simulink subsystem "robotModel"  (R2022b)
settings: Solver=VariableStepAuto  StartTime=0.0  StopTime=10.0  RelTol=1e-3
undefined symbols (not defined in the file or in its folder): DiscIntNeverNeededParam
settings Model: Creator=Wikian  LastModifiedBy=Wikian

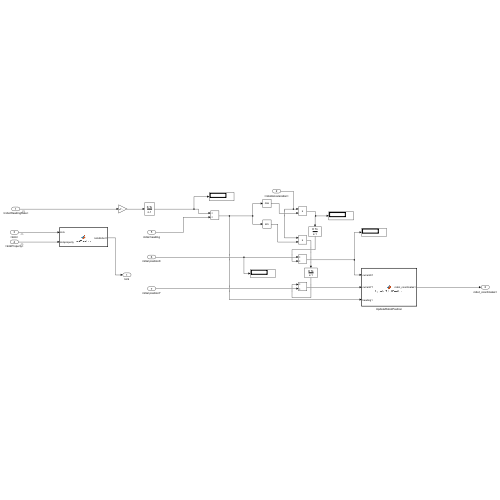
[thumbnail: Simulink's stored preview of the top-level diagram]
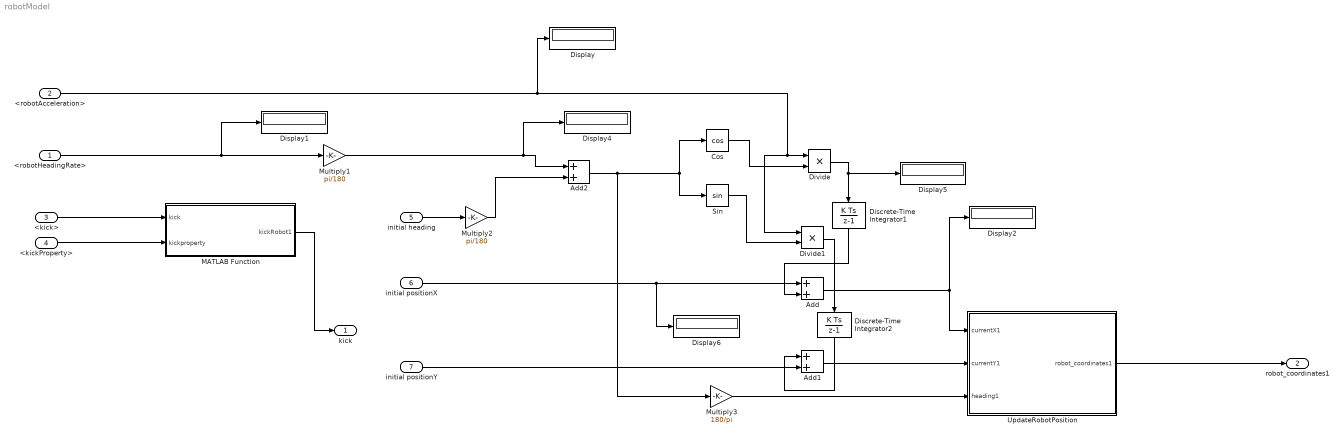
== system robotModel ==
  <robotHeadingRate> : Inport
  <robotAcceleration> : Inport  Port=2
  <kick> : Inport  Port=3
  <kickProperty> : Inport  Port=4
  initial heading : Inport  Port=5
  initial positionX : Inport  Port=6
  initial positionY : Inport  Port=7
  Add : Sum
  Add1 : Sum
  Add2 : Sum
  Cos : Trigonometry  Operator=cos
  Discrete-Time Integrator1 : DiscreteIntegrator  SampleTime=-1  ICPrevOutput=DiscIntNeverNeededParam  ICPrevScaledInput=DiscIntNeverNeededParam
  Discrete-Time Integrator2 : DiscreteIntegrator  SampleTime=-1  ICPrevOutput=DiscIntNeverNeededParam  ICPrevScaledInput=DiscIntNeverNeededParam
  Display{,1..2,4..6} (6 alike) : Display
  Divide : Product  Inputs=**
  Divide1 : Product  Inputs=**
  MATLAB Function : MATLAB Function  TreatAsAtomicUnit=on
  Multiply1 : Gain  Gain=pi/180
  Multiply2 : Gain  Gain=pi/180
  Multiply3 : Gain  Gain=180/pi
  Sin : Trigonometry
  UpdateRobotPosition : MATLAB Function  TreatAsAtomicUnit=on
  kick : Outport
  robot_coordinates1 : Outport  Port=2
  wires:
  Multiply2/1 -> Add2/2
  <robotHeadingRate>/1 -> Display1/1, Multiply1/1
  <kickProperty>/1 -> MATLAB Function/2(kickproperty)
  MATLAB Function/1(kickRobot1) -> kick/1
  <kick>/1 -> MATLAB Function/1(kick)
  Add/1 -> UpdateRobotPosition/1(currentX1), Display2/1
  UpdateRobotPosition/1(robot_coordinates1) -> robot_coordinates1/1
  Add1/1 -> UpdateRobotPosition/2(currentY1)
  initial positionX/1 -> Add/1, Display6/1
  initial positionY/1 -> Add1/2
  Sin/1 -> Divide1/2
  <robotAcceleration>/1 -> Display/1, Divide/1, Divide1/1
  Discrete-Time Integrator1/1 -> Add/2
  Divide1/1 -> Discrete-Time Integrator2/1
  Discrete-Time Integrator2/1 -> Add1/1
  initial heading/1 -> Multiply2/1
  Multiply1/1 -> Display4/1, Add2/1
  Add2/1 -> Cos/1, Sin/1, Multiply3/1
  Cos/1 -> Divide/2
  Divide/1 -> Discrete-Time Integrator1/1, Display5/1
  Multiply3/1 -> UpdateRobotPosition/3(heading1)

== matlab function robotModel/MATLAB Function ==
  data: kick input; kickRobot1 output; kickproperty input
function kickRobot1= kickCombine(kick,kickproperty)

 
    % put heading in vector
    kickRobot1 = [kick, kickproperty];
   
end

== matlab function robotModel/UpdateRobotPosition ==
  data: currentX1 input; robot_coordinates1 output; currentY1 input; heading1 input
function robot_coordinates1  = UpdateRobotPosition(currentX1, currentY1, heading1)

 
    % put heading in vector
    currentPosition = [currentX1, currentY1, heading1];
    
   
    % output the vector
    robot_coordinates1 = currentPosition;
end
